simulink model "control_1"  (R2021b)
settings: Solver=FixedStepDiscrete  StartTime=0.0  StopTime=10.0  RelTol=1e-3
settings Model: Creator=Li Chong  LastModifiedBy=Li Chong
settings OptimizationCC: DefaultParameterBehavior=Inlined  EnhancedBackFolding=on  PassReuseOutputArgsAs=Individual arguments  ZeroExternalMemoryAtStartup=off  ZeroInternalMemoryAtStartup=off  OptimizeBlockOrder=speed  DifferentSizesBufferReuse=on  OptimizationCustomize=off  EfficientTunableParamExpr=on
settings DebuggingCC: ParameterTunabilityLossMsg=error
settings SFSimCC: MATLABDynamicMemAlloc=off
settings RTWCC: Description=Embedded Coder  SystemTargetFile=ert.tlc  TemplateMakefile=ert_default_tmf  GenerateReport=on
settings CodeAppCC: ForceParamTrailComments=on  IgnoreCustomStorageClasses=off  MaxIdLength=64  OperatorAnnotations=on  SimulinkDataObjDesc=on  SFDataObjDesc=on  InsertBlockDesc=on
settings ERTTargetCC: TargetLangStandard=C99 (ISO)  GenerateSampleERTMain=on  InlinedParameterPlacement=NonHierarchical  ERTCustomFileTemplate=example_file_process.tlc

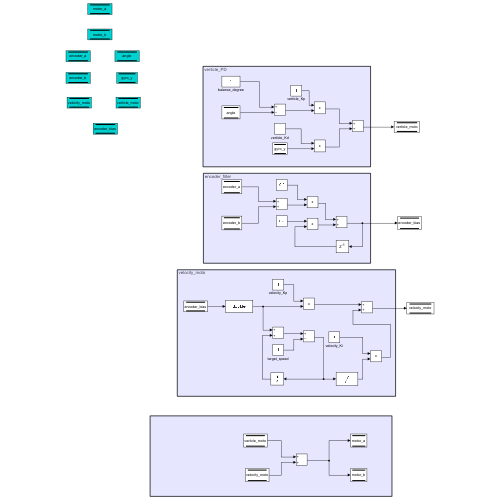
[thumbnail: Simulink's stored preview of the top-level diagram]
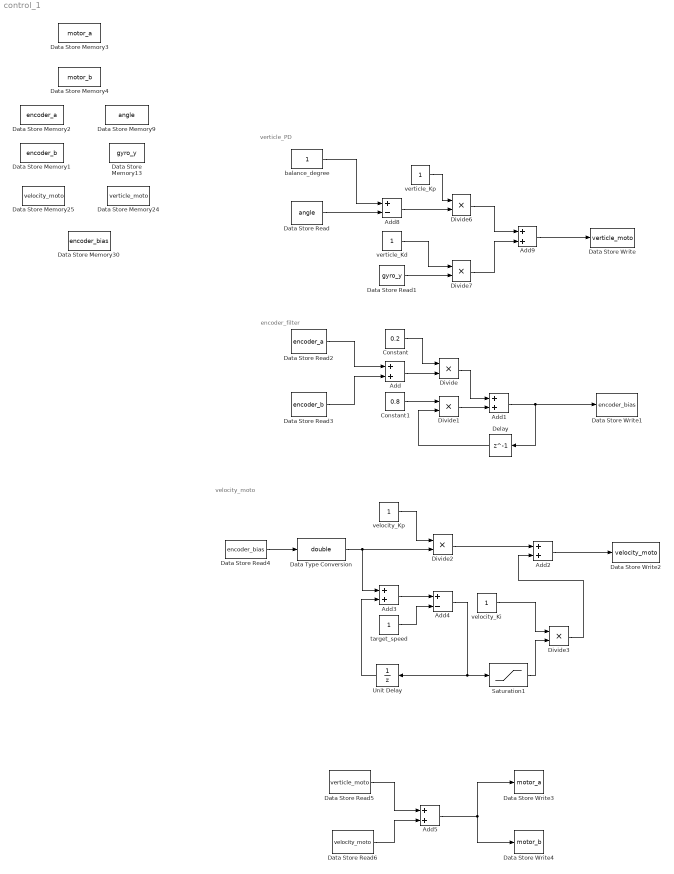
== system control_1 ==
  note: velocity_moto
  note: encoder_filter
  note: verticle_PD
  Add{,1..3,5,9} (6 alike) : Sum
  Add4 : Sum  Inputs=+-
  Add8 : Sum  Inputs=+-
  Constant : Constant  Value=0.2
  Constant1 : Constant  Value=0.8
  Data Store Memory1 : DataStoreMemory  DataStoreName=encoder_b  ReadBeforeWriteMsg=warning  WriteAfterWriteMsg=warning  WriteAfterReadMsg=warning  ShowAdditionalParam=off  OutDataTypeStr=int16
  Data Store Memory13 : DataStoreMemory  DataStoreName=gyro_y  ReadBeforeWriteMsg=warning  WriteAfterWriteMsg=warning  WriteAfterReadMsg=warning  ShowAdditionalParam=off  OutDataTypeStr=double
  Data Store Memory2 : DataStoreMemory  DataStoreName=encoder_a  ReadBeforeWriteMsg=warning  WriteAfterWriteMsg=warning  WriteAfterReadMsg=warning  ShowAdditionalParam=off  OutDataTypeStr=int16
  Data Store Memory24 : DataStoreMemory  DataStoreName=verticle_moto  ReadBeforeWriteMsg=warning  WriteAfterWriteMsg=warning  WriteAfterReadMsg=warning  ShowAdditionalParam=off
  Data Store Memory25 : DataStoreMemory  DataStoreName=velocity_moto  ReadBeforeWriteMsg=warning  WriteAfterWriteMsg=warning  WriteAfterReadMsg=warning  ShowAdditionalParam=off
  Data Store Memory3 : DataStoreMemory  DataStoreName=motor_a  ReadBeforeWriteMsg=warning  WriteAfterWriteMsg=warning  WriteAfterReadMsg=warning  ShowAdditionalParam=off  OutDataTypeStr=double
  Data Store Memory30 : DataStoreMemory  DataStoreName=encoder_bias  ReadBeforeWriteMsg=warning  WriteAfterWriteMsg=warning  WriteAfterReadMsg=warning  ShowAdditionalParam=off  OutDataTypeStr=double
  Data Store Memory4 : DataStoreMemory  DataStoreName=motor_b  ReadBeforeWriteMsg=warning  WriteAfterWriteMsg=warning  WriteAfterReadMsg=warning  ShowAdditionalParam=off  OutDataTypeStr=double
  Data Store Memory9 : DataStoreMemory  DataStoreName=angle  ReadBeforeWriteMsg=warning  WriteAfterWriteMsg=warning  WriteAfterReadMsg=warning  ShowAdditionalParam=off  OutDataTypeStr=double
  Data Store Read : DataStoreRead  DataStoreName=angle  IndexOptions=Index vector (dialog)  Indices=1  OutputSizes=1
  Data Store Read1 : DataStoreRead  DataStoreName=gyro_y  IndexOptions=Index vector (dialog)  Indices=1  OutputSizes=1
  Data Store Read2 : DataStoreRead  DataStoreName=encoder_a  IndexOptions=Index vector (dialog)  Indices=1  OutputSizes=1
  Data Store Read3 : DataStoreRead  DataStoreName=encoder_b  IndexOptions=Index vector (dialog)  Indices=1  OutputSizes=1
  Data Store Read4 : DataStoreRead  DataStoreName=encoder_bias  IndexOptions=Index vector (dialog)  Indices=1  OutputSizes=1
  Data Store Read5 : DataStoreRead  DataStoreName=verticle_moto  IndexOptions=Index vector (dialog)  Indices=1  OutputSizes=1
  Data Store Read6 : DataStoreRead  DataStoreName=velocity_moto  IndexOptions=Index vector (dialog)  Indices=1  OutputSizes=1
  Data Store Write : DataStoreWrite  DataStoreName=verticle_moto  IndexOptions=Index vector (dialog)  Indices=1  OutputSizes=1
  Data Store Write1 : DataStoreWrite  DataStoreName=encoder_bias  IndexOptions=Index vector (dialog)  Indices=1  OutputSizes=1
  Data Store Write2 : DataStoreWrite  DataStoreName=velocity_moto  IndexOptions=Index vector (dialog)  Indices=1  OutputSizes=1
  Data Store Write3 : DataStoreWrite  DataStoreName=motor_a  IndexOptions=Index vector (dialog)  Indices=1  OutputSizes=1
  Data Store Write4 : DataStoreWrite  DataStoreName=motor_b  IndexOptions=Index vector (dialog)  Indices=1  OutputSizes=1
  Data Type Conversion : DataTypeConversion  OutDataTypeStr=double
  Delay : Delay  DelayLength=1  InitialCondition=0
  Divide{,1..3,6..7} (6 alike) : Product  Inputs=**
  Saturation1 : Saturate  UpperLimit=10000  LowerLimit=-10000
  Unit Delay : UnitDelay  SampleTime=-1  HasFrameUpgradeWarning=on
  balance_degree : Constant
  target_speed : Constant
  velocity_Ki : Constant
  velocity_Kp : Constant
  verticle_Kd : Constant
  verticle_Kp : Constant
  wires:
  velocity_Kp/1 -> Divide2/1
  Data Type Conversion/1 -> Add3/1, Divide2/2
  Divide2/1 -> Add2/1
  Unit Delay/1 -> Add3/2
  Saturation1/1 -> Divide3/2
  Divide3/1 -> Add2/2
  Add3/1 -> Add4/1
  target_speed/1 -> Add4/2
  Add4/1 -> Saturation1/1, Unit Delay/1
  velocity_Ki/1 -> Divide3/1
  Data Store Read/1 -> Add8/2
  balance_degree/1 -> Add8/1
  Add8/1 -> Divide6/2
  verticle_Kp/1 -> Divide6/1
  Data Store Read1/1 -> Divide7/2
  verticle_Kd/1 -> Divide7/1
  Divide6/1 -> Add9/1
  Divide7/1 -> Add9/2
  Add9/1 -> Data Store Write/1
  Constant1/1 -> Divide1/1
  Divide1/1 -> Add1/2
  Constant/1 -> Divide/1
  Add1/1 -> Delay/1, Data Store Write1/1
  Divide/1 -> Add1/1
  Add/1 -> Divide/2
  Data Store Read3/1 -> Add/2
  Data Store Read2/1 -> Add/1
  Delay/1 -> Divide1/2
  Data Store Read4/1 -> Data Type Conversion/1
  Add2/1 -> Data Store Write2/1
  Add5/1 -> Data Store Write3/1, Data Store Write4/1
  Data Store Read5/1 -> Add5/1
  Data Store Read6/1 -> Add5/2
